simulink model "test_LQR_x1d"  (R2023a)
settings: Solver=VariableStepAuto  StartTime=0.0  StopTime=10  RelTol=1e-3
values from neighbouring files (symbols this model uses):
  k1 = K(1)    [test_LQR.m]
  k2 = K(2)    [test_LQR.m]
settings Model: Creator=z'k'x  LastModifiedBy=z'k'x

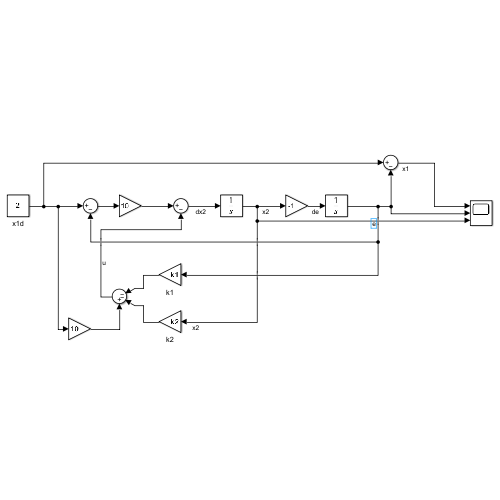
[thumbnail: Simulink's stored preview of the top-level diagram]
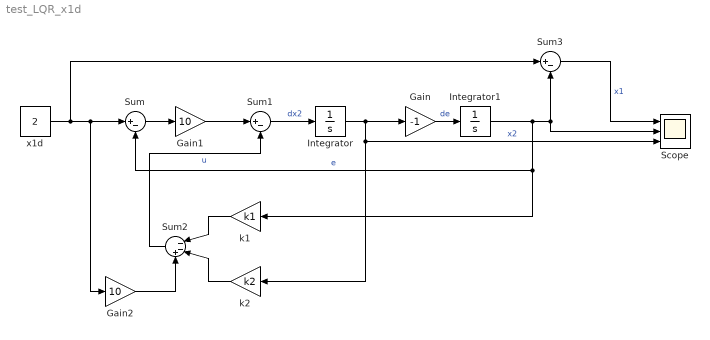
== system test_LQR_x1d ==
  Gain : Gain  Gain=-1
  Gain1 : Gain  Gain=10
  Gain2 : Gain  Gain=10
  Integrator : Integrator  InitialCondition=1
  Integrator1 : Integrator  InitialCondition=5
  Scope : Scope  NumInputPorts=3
  Sum : Sum  Inputs=|+-
  Sum1 : Sum  Inputs=|+-
  Sum2 : Sum  Inputs=|--+
  Sum3 : Sum  Inputs=|+-
  k1 : Gain  Gain=k1
  k2 : Gain  Gain=k2
  x1d : Constant  Value=2
  wires:
  Integrator/1 -> Gain/1, k2/1, Scope/3  "x2"
  Integrator1/1 -> Sum3/2, Scope/2, k1/1, Sum/2  "e"
  Sum/1 -> Gain1/1
  x1d/1 -> Sum3/1, Gain2/1, Sum/1
  Gain1/1 -> Sum1/1
  k1/1 -> Sum2/1
  k2/1 -> Sum2/2
  Sum1/1 -> Integrator/1  "dx2"
  Gain2/1 -> Sum2/3
  Sum2/1 -> Sum1/2  "u"
  Gain/1 -> Integrator1/1  "de"
  Sum3/1 -> Scope/1  "x1"
